simulink library "pressure_drop_quadratic_fitted_data"  (Simulink 8.2)
settings: Solver=ode45  StartTime=0.0  StopTime=10.0  RelTol=1e-3
undefined symbols (not defined in the file): acol
settings Model: Creator=lena.frank  LastModifiedBy=drhf

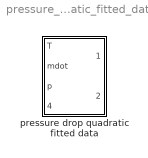
== system pressure_drop_quadratic_fitted_data ==
  pressure drop quadratic fitted data : Subsystem  mask(pressure drop quadratic fitted data, fluid water){b=0.006201*3.6e4, a=0.000096*1.296e9, aonecol=1.96, acol=acol}
      mask prompts: b "linear term of pressure drop in [Pa/(kg/s)]"; a "quadratic term of pressure drop in [Pa/(kg/s)²]"; aonecol "surface of one collector element in [m²]"; acol "total surface of array (DO NOT CHANGE HERE)"
      mask help:
      | This block calculates the pressure drop of a collector from a fitted parabolic curve. Other temperatures than at test condition are not corrected.
      | Give parameters in SI-units.
      | Multiply with 3.6e5 to convert from [mbar/(l/h)] to [Pa/(kg/s)].
      | Multiply with 1.296e9 to convert from [mbar/(l/h)²] to [Pa/(kg/s)²].
      | Set "surface of one collector" to the surface of one collector for a parallel arrangement of collectors. Set it to the surface of the array "acol" to model a series arrangement.
      mask Help: web(fullfile(path_carnot('help'),'pressure_drop_quadratic_fitted_data.html'),'-helpbrowser')

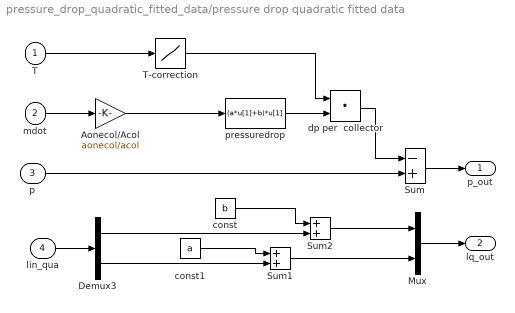
== system pressure_drop_quadratic_fitted_data/pressure drop quadratic fitted data ==
  T : Inport
  mdot : Inport  Port=2
  p : Inport  Port=3
  lin_qua : Inport  Port=4
  Aonecol/Acol : Gain  Gain=aonecol/acol  SaturateOnIntegerOverflow=on  OutDataTypeStr=Inherit: Same as input  ParamDataTypeStr=Inherit: Same as input
  Demux3 : Demux  Outputs=2
  Mux : Mux  Inputs=2
  Sum : Sum  Inputs=-+  SaturateOnIntegerOverflow=on  InputSameDT=on  OutDataTypeStr=Inherit: Same as first input
  Sum1 : Sum  SaturateOnIntegerOverflow=on  InputSameDT=on  OutDataTypeStr=Inherit: Same as first input
  Sum2 : Sum  SaturateOnIntegerOverflow=on  InputSameDT=on  OutDataTypeStr=Inherit: Same as first input
  T-correction : Lookup  InputValues=[0 400]  Table=[1 1]  SaturateOnIntegerOverflow=on
  const : Constant  Value=b
  const1 : Constant  Value=a
  dp per  collector : DotProduct  OutDataTypeStr=Inherit: Inherit via internal rule
  pressuredrop : Fcn  Expr=(a*u[1]+b)*u[1]
  p_out : Outport
  lq_out : Outport  Port=2
  wires:
  pressuredrop/1 -> dp per  collector/2
  T-correction/1 -> dp per  collector/1
  lin_qua/1 -> Demux3/1
  Demux3/2 -> Sum1/2
  Mux/1 -> lq_out/1
  p/1 -> Sum/2
  dp per  collector/1 -> Sum/1
  Sum/1 -> p_out/1
  Sum1/1 -> Mux/2
  Demux3/1 -> Sum2/2
  const/1 -> Sum2/1
  const1/1 -> Sum1/1
  Sum2/1 -> Mux/1
  T/1 -> T-correction/1
  Aonecol/Acol/1 -> pressuredrop/1
  mdot/1 -> Aonecol/Acol/1
